simulink model "EPT"  (R2019b)
settings: Solver=FixedStepDiscrete  StartTime=0.0  StopTime=5  FixedStep=0.005  RelTol=1e-3  EnableMultiTasking=on
PreLoadFcn:
  | try, model_open; catch, disp('Error occurred while executing model pre-load callback: model_open.m'); disp('Please assure that the MATLAB working directory is set to the model directory before opening.'); end
InitFcn:
  | try, model_open; catch, end
undefined symbols (not defined in the file or in its folder): Bridge, GCM, H, ln, raptor_get_param_eval, raptor_get_safe_string, raptor_xcp_function
libraries: Raptor_lib x2810, simulink x374, hdlsllib x19
(part 39 of 45)

== system EPT/Foreground_TimeBase_5ms/CAN/CAN2_exec/ECHS/EPT2ECHS_TX/100ms_exec/0x1852FFF4_DBC ==
  note: Read_Actual_Torque
  Trigger : TriggerPort  VariantControl=Variant  PortDimensions=1
  Abs : Abs
  Constant : Constant  Value=8  OutDataTypeStr=uint8
  Constant1 : Constant  Value=0.01
  Constant2 : Constant  Value=0.02
  Convert_Data2Byte : Subsystem
  Convert_Data2Byte1 : Subsystem
  Data Type Conversion{,2..3,7..10} (7 alike) : DataTypeConversion
  Data Type Conversion{1,4..6} (4 alike) : DataTypeConversion  OutDataTypeStr=uint8
  Mux : Mux  Inputs=8
  raptor_adjustment7 : Raptor_lib/Data Storage/raptor_adjustment  paramName='EPT2ECHS_IV_TxID'  nameSource=Parameter  initValue=hex2dec('25')  dataType=uint32  storage=Calibration  calDispType=Number  calEnum={'False', 'True'}  calGain=1.0  calOffset=0.0  calMax=inf  calMin=-inf  calFormat='-1'  calUnit=''  calHelp=''  calAccess=1  calFunction=raptor_xcp_function(gcb)  calDispHeaders=off  calColHeaders={'Col1' 'Col2' 'Col3'}  calRowHeaders={'Row1' 'Row2' 'Row3'}
      settings: SourceProductName=Raptor
  raptor_can_txmsg : Raptor_lib/CAN/raptor_can_txmsg  canDefinition=struct('dbcFile', 'EPTvsECHS_V1.dbc','message', 'Display_Info_G3_Motor_MCU','comment', '','signals', {{'EPT_MOTOR_FAULT','EPT_MCU_OVERTEMP','EPT_MOTOR_OVERTEMP','EPT_MCU_TEMP','EPT_MOTOR_TEMP','EPT_MOTOR_TRQ','EPT_MOTOR_SPD'}},'enabled', [ 1 1 1 1 1 1 1;],'canBus', '''CAN2''','messageID', [ 408092660;],'idMask', [ 536870911;],'payloadMask', [],'payloadValue', [],'period', [ 0;],'mailbox', '','queueSize', [ 1;],'label', [ 1;],'ver', [ 2;],'showID', [ 0;],'showRaw', [ 0;],'fill', [ 0;],'editID', [ 0;],'signalOrder', [ 2;],'signalAscDes', [ 1;])  canBus='CAN2'  queueSize=1  payloadMask=[]  payloadValue=[]  period=0  showID=0  label=1  idMask=hex2dec('1FFFFFFF')  fill=0  id=408092660  showRaw=0  signalOrder=2  signalInfo={{struct('Name', 'EPT_MOTOR_OVERTEMP','Startbit', [ 0;],'SignalSize', [ 1;],'ByteOrder', 'LittleEndian','ValueType', 'UNSIGNED','Class', 'uint8','Signed', [ 0;],'Factor', [ 1;],'Offset', [ 0;],'Min', [ 0;],'Max', [ 0;],'Units', '','Comment', '','StartBit', [ 40;]),struct('Name', 'EPT_MOTOR_FAULT','Startbit', [ 0;],'SignalSize', [ 1;],'ByteOrder', 'LittleEndian','ValueType', 'UNSIGNED','Class', 'uint8','Signed', [ 0;],'Factor', [ 1;],'Offset', [ 0;],'Min', [ 0;],'Max', [ 0;],'Units', '','Comment', '','StartBit', [ 42;]),struct('Name', 'EPT_MCU_OVERTEMP','Startbit', [ 0;],'SignalSize', [ 1;],'ByteOrder', 'LittleEndian','ValueType', 'UNSIGNED','Class', 'uint8','Signed', [ 0;],'Factor', [ 1;],'Offset', [ 0;],'Min', [ 0;],'Max', [ 0;],'Units', '','Comment', '','StartBit', [ 41;]),struct('Name', 'EPT_MOTOR_TRQ','Startbit', [ 0;],'SignalSize', [ 8;],'ByteOrder', 'LittleEndian','ValueType', 'UNSIGNED','Class', 'uint8','Signed', [ 0;],'Factor', [ 0.4;],'Offset', [ 0;],'Min', [ 0;],'Max', [ 0;],'Units', '%','Comment', '','StartBit', [ 16;]),struct('Name', 'EPT_MOTOR_SPD','Startbit', [ 0;],'SignalSize', [ 16;],'ByteOrder', 'LittleEndian','ValueType', 'UNSIGNED','Class', 'uint16','Signed', [ 0;],'Factor', [ 1;],'Offset', [ 0;],'Min', [ 0;],'Max', [ 8000;],'Units', 'rpm','Comment', '','StartBit', [ 0;]),struct('Name', 'EPT_MCU_TEMP','Startbit', [ 0;],'SignalSize', [ 8;],'ByteOrder', 'LittleEndian','ValueType', 'UNSIGNED','Class', 'uint8','Signed', [ 0;],'Factor', [ 1;],'Offset', [ -40;],'Min', [ 0;],'Max', [ 100;],'Units', '℃','Comment', '','StartBit', [ 32;]),struct('Name', 'EPT_MOTOR_TEMP','Startbit', [ 0;],'SignalSize', [ 8;],'ByteOrder', 'LittleEndian','ValueType', 'UNSIGNED','Class', 'uint8','Signed', [ 0;],'Factor', [ 1;],'Offset', [ -40;],'Min', [ 0;],'Max', [ 100;],'Units', '℃','Comment', '','StartBit', [ 24;])}}
      settings: SourceProductName=Raptor
  raptor_can_txraw : Raptor_lib/CAN/raptor_can_txraw  canBus='CAN2'  queueSize=1  showIdTypePort=0  idTypeSelectValues=Standard|Extended  idTypeSelect=Standard
      settings: SourceProductName=Raptor
  raptor_data_def1 : Raptor_lib/Data Storage/raptor_data_def  dataName='EPT_MOTOR_TRQ'  initValue=0  dataType=double  storage=Volatile (RAM)  calVisible=on  calType=Measurement  calDispType=Number  calEnum={'False', 'True'}  calGain=1.0  calOffset=0  calMin=-inf  calMax=inf  calFormat='-1'  calUnit=''  calHelp=''  calAccess=1  calFunction=raptor_xcp_function(gcb)  calDispHeaders=off  calColHeaders={'Col1' 'Col2' 'Col3'}  calRowHeaders={'Row1' 'Row2' 'Row3'}
      settings: SourceProductName=Raptor
  raptor_data_def2 : Raptor_lib/Data Storage/raptor_data_def  dataName='EPT_MOTOR_FAULT'  initValue=0  dataType=boolean  storage=Volatile (RAM)  calVisible=on  calType=Measurement  calDispType=Number  calEnum={'False', 'True'}  calGain=1.0  calOffset=0  calMin=-inf  calMax=inf  calFormat='-1'  calUnit=''  calHelp=''  calAccess=1  calFunction=raptor_xcp_function(gcb)  calDispHeaders=off  calColHeaders={'Col1' 'Col2' 'Col3'}  calRowHeaders={'Row1' 'Row2' 'Row3'}
      settings: SourceProductName=Raptor
  raptor_data_def3 : Raptor_lib/Data Storage/raptor_data_def  dataName='EPT_MOTOR_SPD_DUP'  initValue=0  dataType=double  storage=Volatile (RAM)  calVisible=on  calType=Measurement  calDispType=Number  calEnum={'False', 'True'}  calGain=1.0  calOffset=0  calMin=-inf  calMax=inf  calFormat='-1'  calUnit=''  calHelp=''  calAccess=1  calFunction=raptor_xcp_function(gcb)  calDispHeaders=off  calColHeaders={'Col1' 'Col2' 'Col3'}  calRowHeaders={'Row1' 'Row2' 'Row3'}
      settings: SourceProductName=Raptor
  raptor_data_read1 : Raptor_lib/Data Storage/raptor_data_read  dataName='EPT_BPOBU_CURR'  dataShape=Scalar  idxSource=Input  idxRow=1  idxCol=1
      settings: SourceProductName=Raptor
  raptor_data_read11 : Raptor_lib/Data Storage/raptor_data_read  dataName='EPT_MOTOR_TRQ'  dataShape=Scalar  idxSource=Input  idxRow=1  idxCol=1
      settings: SourceProductName=Raptor
  raptor_data_read2 : Raptor_lib/Data Storage/raptor_data_read  dataName='EPT_MOTOR_SPD_DUP'  dataShape=Scalar  idxSource=Input  idxRow=1  idxCol=1
      settings: SourceProductName=Raptor
  raptor_data_read3 : Raptor_lib/Data Storage/raptor_data_read  dataName='Warning_Temperature_MCU_High'  dataShape=Scalar  idxSource=Input  idxRow=1  idxCol=1
      settings: SourceProductName=Raptor
  raptor_data_read4 : Raptor_lib/Data Storage/raptor_data_read  dataName='Fault_Temperature_Motor_High'  dataShape=Scalar  idxSource=Input  idxRow=1  idxCol=1
      settings: SourceProductName=Raptor
  raptor_data_read5 : Raptor_lib/Data Storage/raptor_data_read  dataName='EPT_BPOBU_VOLT'  dataShape=Scalar  idxSource=Input  idxRow=1  idxCol=1
      settings: SourceProductName=Raptor
  raptor_data_read6 : Raptor_lib/Data Storage/raptor_data_read  dataName='Read_Motor_Temp'  dataShape=Scalar  idxSource=Input  idxRow=1  idxCol=1
      settings: SourceProductName=Raptor
  raptor_data_read7 : Raptor_lib/Data Storage/raptor_data_read  dataName='Read_Motor_Speed'  dataShape=Scalar  idxSource=Input  idxRow=1  idxCol=1
      settings: SourceProductName=Raptor
  raptor_data_read8 : Raptor_lib/Data Storage/raptor_data_read  dataName='Read_Controller_Temp'  dataShape=Scalar  idxSource=Input  idxRow=1  idxCol=1
      settings: SourceProductName=Raptor
  raptor_data_read9 : Raptor_lib/Data Storage/raptor_data_read  dataName='EPT_MOTOR_FAULT'  dataShape=Scalar  idxSource=Input  idxRow=1  idxCol=1
      settings: SourceProductName=Raptor
  raptor_data_write17 : Raptor_lib/Data Storage/raptor_data_write  dataName='EPT_MOTOR_SPD_DUP'  dataShape=Scalar  idxSource=Input Port  idxRow=1  idxCol=1
      settings: SourceProductName=Raptor
  wires:
  raptor_data_read6/1 -> Data Type Conversion/1
  raptor_data_read8/1 -> Data Type Conversion3/1
  Mux/1 -> raptor_can_txraw/3
  Convert_Data2Byte/1(HighByte) -> Data Type Conversion1/1
  Convert_Data2Byte/2(LowByte) -> Data Type Conversion6/1
  Constant/1 -> raptor_can_txraw/2
  raptor_adjustment7/1 -> raptor_can_txraw/1
  Convert_Data2Byte1/1(HighByte) -> Data Type Conversion5/1
  Convert_Data2Byte1/2(LowByte) -> Data Type Conversion4/1
  raptor_data_read5/1 -> Convert_Data2Byte/1(Data)
  raptor_data_read1/1 -> Convert_Data2Byte1/1(Data)
  Constant1/1 -> Convert_Data2Byte/2(Factor)
  Constant2/1 -> Convert_Data2Byte1/2(Factor)
  Data Type Conversion1/1 -> Mux/3
  Data Type Conversion4/1 -> Mux/6
  Data Type Conversion5/1 -> Mux/5
  Data Type Conversion6/1 -> Mux/4
  raptor_data_read11/1 -> Data Type Conversion8/1
  Data Type Conversion8/1 -> raptor_can_txmsg/6  "EPT_MOTOR_TRQ"
  Data Type Conversion/1 -> raptor_can_txmsg/5  "EPT_MOTOR_TEMP"
  Abs/1 -> Data Type Conversion7/1
  Data Type Conversion7/1 -> raptor_data_write17/1
  raptor_data_read2/1 -> raptor_can_txmsg/7  "EPT_MOTOR_SPD"
  raptor_data_read7/1 -> Abs/1
  raptor_data_read4/1 -> Data Type Conversion9/1
  raptor_data_read3/1 -> Data Type Conversion2/1
  Data Type Conversion3/1 -> raptor_can_txmsg/4  "EPT_MCU_TEMP"
  Data Type Conversion2/1 -> raptor_can_txmsg/2  "EPT_MCU_OVERTEMP"
  Data Type Conversion9/1 -> raptor_can_txmsg/3  "EPT_MOTOR_OVERTEMP"
  Data Type Conversion10/1 -> raptor_can_txmsg/1  "EPT_MOTOR_FAULT"
  raptor_data_read9/1 -> Data Type Conversion10/1

== system EPT/Foreground_TimeBase_5ms/CAN/CAN2_exec/ECHS/EPT2ECHS_TX/100ms_exec/0x1853FFF4_DBC ==
  Trigger : TriggerPort  VariantControl=Variant  PortDimensions=1
  raptor_can_txmsg : Raptor_lib/CAN/raptor_can_txmsg  canDefinition=struct('dbcFile', 'EPTvsECHS_V1.dbc','message', 'Display_Info_G4_ESS_BPSWU','comment', '','signals', {{'EPT_PWCU_FAULT','EPT_BPSWU_SWAP_RMND','EPT_BPSWU_STA','EPT_PWCU_OUT_PWR','EPT_PWCU_TEMP','EPT_BPSWU_SOC','EPT_BPSWU_FCAP','EPT_BPSWU_NUM'}},'enabled', [ 1 1 1 1 1 1 1 1;],'canBus', '''CAN2''','messageID', [ 408158196;],'idMask', [ 536870911;],'payloadMask', [],'payloadValue', [],'period', [ 0;],'mailbox', '','queueSize', [ 1;],'label', [ 1;],'ver', [ 2;],'showID', [ 0;],'showRaw', [ 0;],'fill', [ 0;],'editID', [ 0;],'signalOrder', [ 2;],'signalAscDes', [ 1;])  canBus='CAN2'  queueSize=1  payloadMask=[]  payloadValue=[]  period=0  showID=0  label=1  idMask=hex2dec('1FFFFFFF')  fill=0  id=408158196  showRaw=0  signalOrder=2  signalInfo={{struct('Name', 'EPT_PWCU_TEMP','Startbit', [ 0;],'SignalSize', [ 8;],'ByteOrder', 'LittleEndian','ValueType', 'UNSIGNED','Class', 'uint8','Signed', [ 0;],'Factor', [ 1;],'Offset', [ -40;],'Min', [ 0;],'Max', [ 0;],'Units', '°C','Comment', '','StartBit', [ 24;]),struct('Name', 'EPT_PWCU_OUT_PWR','Startbit', [ 0;],'SignalSize', [ 8;],'ByteOrder', 'LittleEndian','ValueType', 'UNSIGNED','Class', 'uint8','Signed', [ 0;],'Factor', [ 0.1;],'Offset', [ 0;],'Min', [ 0;],'Max', [ 0;],'Units', 'Kw','Comment', '','StartBit', [ 32;]),struct('Name', 'EPT_PWCU_FAULT','Startbit', [ 0;],'SignalSize', [ 1;],'ByteOrder', 'LittleEndian','ValueType', 'UNSIGNED','Class', 'uint8','Signed', [ 0;],'Factor', [ 1;],'Offset', [ 0;],'Min', [ 0;],'Max', [ 0;],'Units', '','Comment', '','StartBit', [ 48;]),struct('Name', 'EPT_BPSWU_SWAP_RMND','Startbit', [ 0;],'SignalSize', [ 4;],'ByteOrder', 'LittleEndian','ValueType', 'UNSIGNED','Class', 'uint8','Signed', [ 0;],'Factor', [ 1;],'Offset', [ 0;],'Min', [ 0;],'Max', [ 0;],'Units', '','Comment', '','StartBit', [ 44;]),struct('Name', 'EPT_BPSWU_STA','Startbit', [ 0;],'SignalSize', [ 4;],'ByteOrder', 'LittleEndian','ValueType', 'UNSIGNED','Class', 'uint8','Signed', [ 0;],'Factor', [ 1;],'Offset', [ 0;],'Min', [ 0;],'Max', [ 0;],'Units', '','Comment', '','StartBit', [ 40;]),struct('Name', 'EPT_BPSWU_SOC','Startbit', [ 0;],'SignalSize', [ 8;],'ByteOrder', 'LittleEndian','ValueType', 'UNSIGNED','Class', 'uint8','Signed', [ 0;],'Factor', [ 0.5;],'Offset', [ 0;],'Min', [ 0;],'Max', [ 0;],'Units', '%','Comment', '','StartBit', [ 16;]),struct('Name', 'EPT_BPSWU_NUM','Startbit', [ 0;],'SignalSize', [ 4;],'ByteOrder', 'LittleEndian','ValueType', 'UNSIGNED','Class', 'uint8','Signed', [ 0;],'Factor', [ 1;],'Offset', [ 0;],'Min', [ 0;],'Max', [ 0;],'Units', '','Comment', '','StartBit', [ 0;]),struct('Name', 'EPT_BPSWU_FCAP','Startbit', [ 0;],'SignalSize', [ 8;],'ByteOrder', 'LittleEndian','ValueType', 'UNSIGNED','Class', 'uint8','Signed', [ 0;],'Factor', [ 0.4;],'Offset', [ 0;],'Min', [ 0;],'Max', [ 0;],'Units', '%','Comment', '','StartBit', [ 8;])}}
      settings: SourceProductName=Raptor

== system EPT/Foreground_TimeBase_5ms/CAN/CAN2_exec/ECHS/EPT2ECHS_TX/100ms_exec/CountTrigger ==
  Counter : Inport
  Constant1 : Constant  Value=0
  Constant3 : Constant
  CycleTrigger : Subsystem
  Switch : Switch  Threshold=1
  Unit Delay : UnitDelay  SampleTime=-1  HasFrameUpgradeWarning=on
  Tirgger : Outport  VectorParamsAs1DForOutWhenUnconnected=off
  wires:
  Unit Delay/1 -> Switch/2
  CycleTrigger/1(Trigger) -> Unit Delay/1, Tirgger/1
  Counter/1 -> CycleTrigger/2(In2)
  Constant1/1 -> Switch/1
  Constant3/1 -> Switch/3
  Switch/1 -> CycleTrigger/1(In1)

== system EPT/Foreground_TimeBase_5ms/CAN/CAN2_exec/ECHS/EPT2ECHS_TX/10ms_exec/0xC10D0F4_DBC ==
  note: Notes :
      | -EPT 2 ECHS Mode Enable
  Data Type Conversion1 : DataTypeConversion
  EPT_BPOBU_STA : Subsystem
  EPT_EW : Subsystem
  EPT_VEH_MODE_STA : Subsystem
  raptor_can_txmsg : Raptor_lib/CAN/raptor_can_txmsg  canDefinition=struct('dbcFile', 'EPTvsECHS_V1.dbc','message', 'EPT_Feedback_Status','comment', '','signals', {{'EPT_STATUS','EPT_VEH_MODE_STA','EPT_ERROR','EPT_BPOBU_STA','EPT_MAX_DRV_TRQ','EPT_MAX_REG_TRQ','EPT_CONSUMED_WH','EPT_MOTOR_SPD','EPT_GEAR_STA','EPT_CHG_REQ'}},'enabled', [ 1 1 1 1 1 1 1 1 1 1;],'canBus', '''CAN2''','messageID', [ 202428660;],'idMask', [ 536870911;],'payloadMask', [],'payloadValue', [],'period', [ 0;],'mailbox', '','queueSize', [ 1;],'label', [ 1;],'ver', [ 2;],'showID', [ 0;],'showRaw', [ 0;],'fill', [ 0;],'editID', [ 0;],'signalOrder', [ 2;])  canBus='CAN2'  queueSize=1  payloadMask=[]  payloadValue=[]  period=0  showID=0  label=1  idMask=hex2dec('1FFFFFFF')  fill=0  id=202428660  showRaw=0  signalOrder=2  signalInfo={{struct('Name', 'EPT_CHG_REQ','Startbit', [ 0;],'SignalSize', [ 1;],'ByteOrder', 'LittleEndian','ValueType', 'UNSIGNED','Class', 'uint8','Signed', [ 0;],'Factor', [ 1;],'Offset', [ 0;],'Min', [ 0;],'Max', [ 0;],'Units', '','Comment', '','StartBit', [ 63;]),struct('Name', 'EPT_BPOBU_STA','Startbit', [ 0;],'SignalSize', [ 3;],'ByteOrder', 'LittleEndian','ValueType', 'UNSIGNED','Class', 'uint8','Signed', [ 0;],'Factor', [ 1;],'Offset', [ 0;],'Min', [ 0;],'Max', [ 0;],'Units', '','Comment', '','StartBit', [ 5;]),struct('Name', 'EPT_GEAR_STA','Startbit', [ 0;],'SignalSize', [ 4;],'ByteOrder', 'LittleEndian','ValueType', 'UNSIGNED','Class', 'uint8','Signed', [ 0;],'Factor', [ 1;],'Offset', [ 0;],'Min', [ 0;],'Max', [ 0;],'Units', '','Comment', '','StartBit', [ 56;]),struct('Name', 'EPT_CONSUMED_WH','Startbit', [ 0;],'SignalSize', [ 16;],'ByteOrder', 'LittleEndian','ValueType', 'UNSIGNED','Class', 'uint16','Signed', [ 0;],'Factor', [ 1;],'Offset', [ 0;],'Min', [ 0;],'Max', [ 0;],'Units', 'WH','Comment', '','StartBit', [ 24;]),struct('Name', 'EPT_MAX_REG_TRQ','Startbit', [ 0;],'SignalSize', [ 8;],'ByteOrder', 'LittleEndian','ValueType', 'UNSIGNED','Class', 'uint8','Signed', [ 0;],'Factor', [ 1;],'Offset', [ 0;],'Min', [ 0;],'Max', [ 150;],'Units', 'Nm','Comment', '','StartBit', [ 16;]),struct('Name', 'EPT_MOTOR_SPD','Startbit', [ 0;],'SignalSize', [ 16;],'ByteOrder', 'LittleEndian','ValueType', 'UNSIGNED','Class', 'uint16','Signed', [ 0;],'Factor', [ 1;],'Offset', [ -12000;],'Min', [ -12000;],'Max', [ 12000;],'Units', 'rpm','Comment', '','StartBit', [ 40;]),struct('Name', 'EPT_STATUS','Startbit', [ 0;],'SignalSize', [ 1;],'ByteOrder', 'LittleEndian','ValueType', 'UNSIGNED','Class', 'uint8','Signed', [ 0;],'Factor', [ 1;],'Offset', [ 0;],'Min', [ 0;],'Max', [ 0;],'Units', '','Comment', '','StartBit', [ 0;]),struct('Name', 'EPT_VEH_MODE_STA','Startbit', [ 0;],'SignalSize', [ 2;],'ByteOrder', 'LittleEndian','ValueType', 'UNSIGNED','Class', 'uint8','Signed', [ 0;],'Factor', [ 1;],'Offset', [ 0;],'Min', [ 0;],'Max', [ 0;],'Units', '','Comment', '','StartBit', [ 1;]),struct('Name', 'EPT_ERROR','Startbit', [ 0;],'SignalSize', [ 2;],'ByteOrder', 'LittleEndian','ValueType', 'UNSIGNED','Class', 'uint8','Signed', [ 0;],'Factor', [ 1;],'Offset', [ 0;],'Min', [ 0;],'Max', [ 0;],'Units', '','Comment', '','StartBit', [ 3;]),struct('Name', 'EPT_MAX_DRV_TRQ','Startbit', [ 0;],'SignalSize', [ 8;],'ByteOrder', 'LittleEndian','ValueType', 'UNSIGNED','Class', 'uint8','Signed', [ 0;],'Factor', [ 1;],'Offset', [ 0;],'Min', [ 0;],'Max', [ 150;],'Units', 'Nm','Comment', '','StartBit', [ 8;])}}
      settings: SourceProductName=Raptor
  raptor_data_def1 : Raptor_lib/Data Storage/raptor_data_def  dataName='EPT_READY'  initValue=0  dataType=uint8  storage=Volatile (RAM)  calVisible=on  calType=Measurement  calDispType=Number  calEnum={'False', 'True'}  calGain=1.0  calOffset=0  calMin=-inf  calMax=inf  calFormat='-1'  calUnit=''  calHelp=''  calAccess=1  calFunction=raptor_xcp_function(gcb)  calDispHeaders=off  calColHeaders={'Col1' 'Col2' 'Col3'}  calRowHeaders={'Row1' 'Row2' 'Row3'}
      settings: SourceProductName=Raptor
  raptor_data_def2 : Raptor_lib/Data Storage/raptor_data_def  dataName='EPT_EW'  initValue=0  dataType=uint8  storage=Volatile (RAM)  calVisible=on  calType=Measurement  calDispType=Number  calEnum={'False', 'True'}  calGain=1.0  calOffset=0  calMin=-inf  calMax=inf  calFormat='-1'  calUnit=''  calHelp=''  calAccess=1  calFunction=raptor_xcp_function(gcb)  calDispHeaders=off  calColHeaders={'Col1' 'Col2' 'Col3'}  calRowHeaders={'Row1' 'Row2' 'Row3'}
      settings: SourceProductName=Raptor
  raptor_data_def3 : Raptor_lib/Data Storage/raptor_data_def  dataName='EPT_MAX_REG_TRQ'  initValue=0  dataType=double  storage=Volatile (RAM)  calVisible=on  calType=Measurement  calDispType=Number  calEnum={'False', 'True'}  calGain=1.0  calOffset=0  calMin=-inf  calMax=inf  calFormat='-1'  calUnit=''  calHelp=''  calAccess=1  calFunction=raptor_xcp_function(gcb)  calDispHeaders=off  calColHeaders={'Col1' 'Col2' 'Col3'}  calRowHeaders={'Row1' 'Row2' 'Row3'}
      settings: SourceProductName=Raptor
  raptor_data_def33 : Raptor_lib/Data Storage/raptor_data_def  dataName='EPT_VEH_MODE_STA'  initValue=0  dataType=uint8  storage=Volatile (RAM)  calVisible=on  calType=Measurement  calDispType=Number  calEnum={'False', 'True'}  calGain=1.0  calOffset=0  calMin=-inf  calMax=inf  calFormat='-1'  calUnit=''  calHelp=''  calAccess=1  calFunction=raptor_xcp_function(gcb)  calDispHeaders=off  calColHeaders={'Col1' 'Col2' 'Col3'}  calRowHeaders={'Row1' 'Row2' 'Row3'}
      settings: SourceProductName=Raptor
  raptor_data_def34 : Raptor_lib/Data Storage/raptor_data_def  dataName='EPT_MAX_DRV_TRQ'  initValue=0  dataType=double  storage=Volatile (RAM)  calVisible=on  calType=Measurement  calDispType=Number  calEnum={'False', 'True'}  calGain=1.0  calOffset=0  calMin=-inf  calMax=inf  calFormat='-1'  calUnit=''  calHelp=''  calAccess=1  calFunction=raptor_xcp_function(gcb)  calDispHeaders=off  calColHeaders={'Col1' 'Col2' 'Col3'}  calRowHeaders={'Row1' 'Row2' 'Row3'}
      settings: SourceProductName=Raptor
  raptor_data_def4 : Raptor_lib/Data Storage/raptor_data_def  dataName='EPT_MOTOR_SPD'  initValue=0  dataType=int16  storage=Volatile (RAM)  calVisible=on  calType=Measurement  calDispType=Number  calEnum={'False', 'True'}  calGain=1.0  calOffset=0  calMin=-inf  calMax=inf  calFormat='-1'  calUnit=''  calHelp=''  calAccess=1  calFunction=raptor_xcp_function(gcb)  calDispHeaders=off  calColHeaders={'Col1' 'Col2' 'Col3'}  calRowHeaders={'Row1' 'Row2' 'Row3'}
      settings: SourceProductName=Raptor
  raptor_data_def5 : Raptor_lib/Data Storage/raptor_data_def  dataName='EPT_CONSUMED_WH'  initValue=0  dataType=double  storage=Volatile (RAM)  calVisible=on  calType=Measurement  calDispType=Number  calEnum={'False', 'True'}  calGain=1.0  calOffset=0  calMin=-inf  calMax=inf  calFormat='-1'  calUnit=''  calHelp=''  calAccess=1  calFunction=raptor_xcp_function(gcb)  calDispHeaders=off  calColHeaders={'Col1' 'Col2' 'Col3'}  calRowHeaders={'Row1' 'Row2' 'Row3'}
      settings: SourceProductName=Raptor
  raptor_data_def6 : Raptor_lib/Data Storage/raptor_data_def  dataName='EPT_BPOBU_STA'  initValue=0  dataType=double  storage=Volatile (RAM)  calVisible=on  calType=Measurement  calDispType=Number  calEnum={'False', 'True'}  calGain=1.0  calOffset=0  calMin=-inf  calMax=inf  calFormat='-1'  calUnit=''  calHelp=''  calAccess=1  calFunction=raptor_xcp_function(gcb)  calDispHeaders=off  calColHeaders={'Col1' 'Col2' 'Col3'}  calRowHeaders={'Row1' 'Row2' 'Row3'}
      settings: SourceProductName=Raptor
  raptor_data_def7 : Raptor_lib/Data Storage/raptor_data_def  dataName='EPT_GEAR_STA'  initValue=0  dataType=int16  storage=Volatile (RAM)  calVisible=on  calType=Measurement  calDispType=Number  calEnum={'False', 'True'}  calGain=1.0  calOffset=0  calMin=-inf  calMax=inf  calFormat='-1'  calUnit=''  calHelp=''  calAccess=1  calFunction=raptor_xcp_function(gcb)  calDispHeaders=off  calColHeaders={'Col1' 'Col2' 'Col3'}  calRowHeaders={'Row1' 'Row2' 'Row3'}
      settings: SourceProductName=Raptor
  raptor_data_def8 : Raptor_lib/Data Storage/raptor_data_def  dataName='EPT_CHG_REQ'  initValue=0  dataType=boolean  storage=Volatile (RAM)  calVisible=on  calType=Measurement  calDispType=Number  calEnum={'False', 'True'}  calGain=1.0  calOffset=0  calMin=-inf  calMax=inf  calFormat='-1'  calUnit=''  calHelp=''  calAccess=1  calFunction=raptor_xcp_function(gcb)  calDispHeaders=off  calColHeaders={'Col1' 'Col2' 'Col3'}  calRowHeaders={'Row1' 'Row2' 'Row3'}
      settings: SourceProductName=Raptor
  raptor_data_read1 : Raptor_lib/Data Storage/raptor_data_read  dataName='EPT_READY'  dataShape=Scalar  idxSource=Input  idxRow=1  idxCol=1
      settings: SourceProductName=Raptor
  raptor_data_read10 : Raptor_lib/Data Storage/raptor_data_read  dataName='EPT_GEAR_STA'  dataShape=Scalar  idxSource=Input  idxRow=1  idxCol=1
      settings: SourceProductName=Raptor
  raptor_data_read11 : Raptor_lib/Data Storage/raptor_data_read  dataName='EPT_CHG_REQ'  dataShape=Scalar  idxSource=Input  idxRow=1  idxCol=1
      settings: SourceProductName=Raptor
  raptor_data_read2 : Raptor_lib/Data Storage/raptor_data_read  dataName='EPT_EW'  dataShape=Scalar  idxSource=Input  idxRow=1  idxCol=1
      settings: SourceProductName=Raptor
  raptor_data_read3 : Raptor_lib/Data Storage/raptor_data_read  dataName='EPT_MAX_DRV_TRQ'  dataShape=Scalar  idxSource=Input  idxRow=1  idxCol=1
      settings: SourceProductName=Raptor
  raptor_data_read4 : Raptor_lib/Data Storage/raptor_data_read  dataName='EPT_VEH_MODE_STA'  dataShape=Scalar  idxSource=Input  idxRow=1  idxCol=1
      settings: SourceProductName=Raptor
  raptor_data_read5 : Raptor_lib/Data Storage/raptor_data_read  dataName='EPT_MAX_REG_TRQ'  dataShape=Scalar  idxSource=Input  idxRow=1  idxCol=1
      settings: SourceProductName=Raptor
  raptor_data_read6 : Raptor_lib/Data Storage/raptor_data_read  dataName='EPT_MOTOR_SPD'  dataShape=Scalar  idxSource=Input  idxRow=1  idxCol=1
      settings: SourceProductName=Raptor
  raptor_data_read7 : Raptor_lib/Data Storage/raptor_data_read  dataName='Read_Motor_Speed'  dataShape=Scalar  idxSource=Input  idxRow=1  idxCol=1
      settings: SourceProductName=Raptor
  raptor_data_read8 : Raptor_lib/Data Storage/raptor_data_read  dataName='EPT_CONSUMED_WH'  dataShape=Scalar  idxSource=Input  idxRow=1  idxCol=1
      settings: SourceProductName=Raptor
  raptor_data_read9 : Raptor_lib/Data Storage/raptor_data_read  dataName='EPT_BPOBU_STA'  dataShape=Scalar  idxSource=Input  idxRow=1  idxCol=1
      settings: SourceProductName=Raptor
  raptor_data_write17 : Raptor_lib/Data Storage/raptor_data_write  dataName='EPT_MOTOR_SPD'  dataShape=Scalar  idxSource=Input Port  idxRow=1  idxCol=1
      settings: SourceProductName=Raptor
  wires:
  raptor_data_read10/1 -> raptor_can_txmsg/9  "EPT_GEAR_STA"
  raptor_data_read6/1 -> raptor_can_txmsg/8  "EPT_MOTOR_SPD"
  raptor_data_read8/1 -> raptor_can_txmsg/7  "EPT_CONSUMED_WH"
  raptor_data_read3/1 -> raptor_can_txmsg/5  "EPT_MAX_DRV_TRQ"
  raptor_data_read9/1 -> raptor_can_txmsg/4  "EPT_BPOBU_STA"
  raptor_data_read4/1 -> raptor_can_txmsg/2  "EPT_VEH_MODE_STA"
  raptor_data_read2/1 -> raptor_can_txmsg/3  "EPT_ERROR"
  raptor_data_read5/1 -> raptor_can_txmsg/6  "EPT_MAX_REG_TRQ"
  raptor_data_read1/1 -> raptor_can_txmsg/1  "EPT_STATUS"
  raptor_data_read11/1 -> raptor_can_txmsg/10  "EPT_CHG_REQ"
  raptor_data_read7/1 -> Data Type Conversion1/1
  Data Type Conversion1/1 -> raptor_data_write17/1

== system EPT/Foreground_TimeBase_5ms/CAN/CAN2_exec/ECHS/EPT2ECHS_TX/500ms_exec/0x1820FFF4_DBC ==
  Trigger : TriggerPort  VariantControl=Variant  PortDimensions=1
  raptor_can_txmsg : Raptor_lib/CAN/raptor_can_txmsg  canDefinition=struct('dbcFile', 'EPTvsECHS_V1.dbc','message', 'Remote_DA_Status_G20_ESS_OBU_1','comment', '','signals', {{'BP_OBU_Fault_G5','BP_OBU_Fault_G4','BP_OBU_Fault_G3','BP_OBU_Fault_G2','BP_OBU_Fault_G1','BP_OBU_Warning_G3','BP_OBU_Warning_G2','BP_OBU_Warning_G1'}},'enabled', [ 1 1 1 1 1 1 1 1;],'canBus', '''CAN2''','messageID', [ 404815860;],'idMask', [ 536870911;],'payloadMask', [],'payloadValue', [],'period', [ 0;],'mailbox', '','queueSize', [ 1;],'label', [ 0;],'ver', [ 2;],'showID', [ 0;],'showRaw', [ 0;],'fill', [ 0;],'editID', [ 0;],'signalOrder', [ 2;],'signalAscDes', [ 1;])  canBus='CAN2'  queueSize=1  payloadMask=[]  payloadValue=[]  period=0  showID=0  label=0  idMask=hex2dec('1FFFFFFF')  fill=0  id=404815860  showRaw=0  signalOrder=2  signalInfo={{struct('Name', 'BP_OBU_Warning_G3','Startbit', [ 0;],'SignalSize', [ 8;],'ByteOrder', 'LittleEndian','ValueType', 'UNSIGNED','Class', 'uint8','Signed', [ 0;],'Factor', [ 1;],'Offset', [ 0;],'Min', [ 0;],'Max', [ 0;],'Units', '','Comment', '','StartBit', [ 16;]),struct('Name', 'BP_OBU_Warning_G2','Startbit', [ 0;],'SignalSize', [ 8;],'ByteOrder', 'LittleEndian','ValueType', 'UNSIGNED','Class', 'uint8','Signed', [ 0;],'Factor', [ 1;],'Offset', [ 0;],'Min', [ 0;],'Max', [ 0;],'Units', '','Comment', '','StartBit', [ 8;]),struct('Name', 'BP_OBU_Warning_G1','Startbit', [ 0;],'SignalSize', [ 8;],'ByteOrder', 'LittleEndian','ValueType', 'UNSIGNED','Class', 'uint8','Signed', [ 0;],'Factor', [ 1;],'Offset', [ 0;],'Min', [ 0;],'Max', [ 0;],'Units', '','Comment', '','StartBit', [ 0;]),struct('Name', 'BP_OBU_Fault_G5','Startbit', [ 0;],'SignalSize', [ 8;],'ByteOrder', 'LittleEndian','ValueType', 'UNSIGNED','Class', 'uint8','Signed', [ 0;],'Factor', [ 1;],'Offset', [ 0;],'Min', [ 0;],'Max', [ 0;],'Units', '','Comment', '','StartBit', [ 56;]),struct('Name', 'BP_OBU_Fault_G4','Startbit', [ 0;],'SignalSize', [ 8;],'ByteOrder', 'LittleEndian','ValueType', 'UNSIGNED','Class', 'uint8','Signed', [ 0;],'Factor', [ 1;],'Offset', [ 0;],'Min', [ 0;],'Max', [ 0;],'Units', '','Comment', '','StartBit', [ 48;]),struct('Name', 'BP_OBU_Fault_G3','Startbit', [ 0;],'SignalSize', [ 8;],'ByteOrder', 'LittleEndian','ValueType', 'UNSIGNED','Class', 'uint8','Signed', [ 0;],'Factor', [ 1;],'Offset', [ 0;],'Min', [ 0;],'Max', [ 0;],'Units', '','Comment', '','StartBit', [ 40;]),struct('Name', 'BP_OBU_Fault_G2','Startbit', [ 0;],'SignalSize', [ 8;],'ByteOrder', 'LittleEndian','ValueType', 'UNSIGNED','Class', 'uint8','Signed', [ 0;],'Factor', [ 1;],'Offset', [ 0;],'Min', [ 0;],'Max', [ 0;],'Units', '','Comment', '','StartBit', [ 32;]),struct('Name', 'BP_OBU_Fault_G1','Startbit', [ 0;],'SignalSize', [ 8;],'ByteOrder', 'LittleEndian','ValueType', 'UNSIGNED','Class', 'uint8','Signed', [ 0;],'Factor', [ 1;],'Offset', [ 0;],'Min', [ 0;],'Max', [ 0;],'Units', '','Comment', '','StartBit', [ 24;])}}
      settings: SourceProductName=Raptor
  raptor_data_read1 : Raptor_lib/Data Storage/raptor_data_read  dataName='BP_OBU_Fault_G4'  dataShape=Scalar  idxSource=Input  idxRow=1  idxCol=1
      settings: SourceProductName=Raptor
  raptor_data_read2 : Raptor_lib/Data Storage/raptor_data_read  dataName='BP_OBU_Fault_G3'  dataShape=Scalar  idxSource=Input  idxRow=1  idxCol=1
      settings: SourceProductName=Raptor
  raptor_data_read3 : Raptor_lib/Data Storage/raptor_data_read  dataName='BP_OBU_Fault_G2'  dataShape=Scalar  idxSource=Input  idxRow=1  idxCol=1
      settings: SourceProductName=Raptor
  raptor_data_read4 : Raptor_lib/Data Storage/raptor_data_read  dataName='BP_OBU_Fault_G5'  dataShape=Scalar  idxSource=Input  idxRow=1  idxCol=1
      settings: SourceProductName=Raptor
  raptor_data_read5 : Raptor_lib/Data Storage/raptor_data_read  dataName='BP_OBU_Fault_G1'  dataShape=Scalar  idxSource=Input  idxRow=1  idxCol=1
      settings: SourceProductName=Raptor
  raptor_data_read6 : Raptor_lib/Data Storage/raptor_data_read  dataName='BP_OBU_Warning_G3'  dataShape=Scalar  idxSource=Input  idxRow=1  idxCol=1
      settings: SourceProductName=Raptor
  raptor_data_read7 : Raptor_lib/Data Storage/raptor_data_read  dataName='BP_OBU_Warning_G2'  dataShape=Scalar  idxSource=Input  idxRow=1  idxCol=1
      settings: SourceProductName=Raptor
  raptor_data_read8 : Raptor_lib/Data Storage/raptor_data_read  dataName='BP_OBU_Warning_G1'  dataShape=Scalar  idxSource=Input  idxRow=1  idxCol=1
      settings: SourceProductName=Raptor
  wires:
  raptor_data_read4/1 -> raptor_can_txmsg/1
  raptor_data_read1/1 -> raptor_can_txmsg/2
  raptor_data_read8/1 -> raptor_can_txmsg/8
  raptor_data_read7/1 -> raptor_can_txmsg/7
  raptor_data_read6/1 -> raptor_can_txmsg/6
  raptor_data_read5/1 -> raptor_can_txmsg/5
  raptor_data_read3/1 -> raptor_can_txmsg/4
  raptor_data_read2/1 -> raptor_can_txmsg/3

== system EPT/Foreground_TimeBase_5ms/CAN/CAN2_exec/ECHS/EPT2ECHS_TX/500ms_exec/CountTrigger ==
  Counter : Inport
  Constant1 : Constant  Value=0
  Constant3 : Constant
  CycleTrigger : Subsystem
  Switch : Switch  Threshold=1
  Unit Delay : UnitDelay  SampleTime=-1  HasFrameUpgradeWarning=on
  Tirgger : Outport  VectorParamsAs1DForOutWhenUnconnected=off
  wires:
  Switch/1 -> CycleTrigger/1(In1)
  Constant3/1 -> Switch/3
  Constant1/1 -> Switch/1
  Counter/1 -> CycleTrigger/2(In2)
  CycleTrigger/1(Trigger) -> Tirgger/1, Unit Delay/1
  Unit Delay/1 -> Switch/2

== system EPT/Foreground_TimeBase_5ms/CAN/CAN2_exec/IVT2/Coulomb Counting Method1/20ms/CountTrigger3 ==
  Counter : Inport
  Constant1 : Constant  Value=0
  Constant3 : Constant
  CycleTrigger : Subsystem
  Switch : Switch  Threshold=1
  Unit Delay1 : UnitDelay  SampleTime=-1  HasFrameUpgradeWarning=on
  Unit Delay2 : UnitDelay  SampleTime=-1  HasFrameUpgradeWarning=on
  Tirgger : Outport  VectorParamsAs1DForOutWhenUnconnected=off
  wires:
  Unit Delay2/1 -> Tirgger/1
  Unit Delay1/1 -> CycleTrigger/1(In1)
  CycleTrigger/1(Trigger) -> Unit Delay2/1, Switch/2
  Counter/1 -> CycleTrigger/2(In2)
  Constant1/1 -> Switch/1
  Constant3/1 -> Switch/3
  Switch/1 -> Unit Delay1/1

== system EPT/Foreground_TimeBase_5ms/CAN/CAN2_exec/IVT2/Coulomb Counting Method1/CountTrigger/CycleTrigger ==
  In1 : Inport
  In2 : Inport  Port=2
  Add : Sum
  Add2 : Sum  Inputs=+-
  Constant2 : Constant  Value=0
  Constant3 : Constant
  Data Type Conversion1 : DataTypeConversion
  Data Type Conversion2 : DataTypeConversion
  Relational Operator1 : RelationalOperator  OutDataTypeStr=boolean  RndMeth=Simplest
  Scope1 : Scope
  Scope2 : Scope
  Switch : Switch  Threshold=1
  Unit Delay : UnitDelay  SampleTime=-1  HasFrameUpgradeWarning=on
  Trigger : Outport  VectorParamsAs1DForOutWhenUnconnected=off
  wires:
  Constant3/1 -> Add2/2
  In2/1 -> Add2/1
  Add2/1 -> Data Type Conversion1/1
  Data Type Conversion2/1 -> Switch/2, Add/2
  Constant2/1 -> Switch/3
  Data Type Conversion1/1 -> Relational Operator1/2
  Relational Operator1/1 -> Trigger/1, Scope2/1
  Switch/1 -> Unit Delay/1, Scope1/1, Relational Operator1/1
  Unit Delay/1 -> Add/1
  In1/1 -> Data Type Conversion2/1
  Add/1 -> Switch/1

== system EPT/Foreground_TimeBase_5ms/CAN/CAN3_exec/OBC/OBC/OBC_Rx/Convert_Byte2Data1 ==
  HighByte : Inport
  LowByte : Inport  Port=2
  Offset : Inport  Port=3
  Factor : Inport  Port=4
  Add2 : Sum
  Add5 : Sum
  Constant10 : Constant  Value=256
  Data Type Conversion10 : DataTypeConversion  OutDataTypeStr=double
  Divide6 : Product  Inputs=**
  Divide9 : Product  Inputs=**
  Data : Outport  VectorParamsAs1DForOutWhenUnconnected=off
  wires:
  Divide6/1 -> Add2/2
  LowByte/1 -> Add2/1
  Add5/1 -> Data Type Conversion10/1
  HighByte/1 -> Divide6/1
  Constant10/1 -> Divide6/2
  Divide9/1 -> Add5/1
  Add2/1 -> Divide9/1
  Data Type Conversion10/1 -> Data/1
  Factor/1 -> Divide9/2
  Offset/1 -> Add5/2

== system EPT/Foreground_TimeBase_5ms/CAN/CAN3_exec/OBC/OBC/OBC_Rx/Convert_Byte2Data2 ==
  HighByte : Inport
  LowByte : Inport  Port=2
  Offset : Inport  Port=3
  Factor : Inport  Port=4
  Add2 : Sum
  Add5 : Sum
  Constant10 : Constant  Value=256
  Data Type Conversion10 : DataTypeConversion  OutDataTypeStr=double
  Divide6 : Product  Inputs=**
  Divide9 : Product  Inputs=**
  Data : Outport  VectorParamsAs1DForOutWhenUnconnected=off
  wires:
  Divide6/1 -> Add2/2
  LowByte/1 -> Add2/1
  Add5/1 -> Data Type Conversion10/1
  HighByte/1 -> Divide6/1
  Constant10/1 -> Divide6/2
  Divide9/1 -> Add5/1
  Add2/1 -> Divide9/1
  Data Type Conversion10/1 -> Data/1
  Factor/1 -> Divide9/2
  Offset/1 -> Add5/2

== system EPT/Foreground_TimeBase_5ms/CAN/CAN3_exec/OBC/OBC/OBC_Rx/Convert_Byte2Data3 ==
  HighByte : Inport
  LowByte : Inport  Port=2
  Offset : Inport  Port=3
  Factor : Inport  Port=4
  Add2 : Sum
  Add5 : Sum
  Constant10 : Constant  Value=256
  Data Type Conversion10 : DataTypeConversion  OutDataTypeStr=double
  Divide6 : Product  Inputs=**
  Divide9 : Product  Inputs=**
  Data : Outport  VectorParamsAs1DForOutWhenUnconnected=off
  wires:
  Divide6/1 -> Add2/2
  LowByte/1 -> Add2/1
  Add5/1 -> Data Type Conversion10/1
  HighByte/1 -> Divide6/1
  Constant10/1 -> Divide6/2
  Divide9/1 -> Add5/1
  Add2/1 -> Divide9/1
  Data Type Conversion10/1 -> Data/1
  Factor/1 -> Divide9/2
  Offset/1 -> Add5/2

== system EPT/Foreground_TimeBase_5ms/CAN/CAN3_exec/OBC/OBC/OBC_Tx/Convert_Data2Byte ==
  Data : Inport
  Factor : Inport  Port=2
  Offset : Inport  Port=3
  Add1 : Sum
  Bitwise Operator : simulink/Logic and Bit Operations/Bitwise Operator  logicop=AND  UseBitMask=on  BitMask=bin2dec('1111111100000000')  BitMaskRealWorld=Stored Integer
  Bitwise Operator1 : simulink/Logic and Bit Operations/Bitwise Operator  logicop=AND  UseBitMask=on  BitMask=bin2dec('0000000011111111')  BitMaskRealWorld=Stored Integer
  Constant : Constant
  Data Type Conversion1 : DataTypeConversion  OutDataTypeStr=uint16
  Divide1 : Product  Inputs=*/
  Divide2 : Product  Inputs=**
  Shift Arithmetic : ArithShift  BitShiftNumber=8  BitShiftDirection=Right
  HighByte : Outport  VectorParamsAs1DForOutWhenUnconnected=off
  LowByte : Outport  Port=2  VectorParamsAs1DForOutWhenUnconnected=off
  wires:
  Divide2/1 -> Data Type Conversion1/1
  Data/1 -> Add1/1
  Add1/1 -> Divide2/1
  Data Type Conversion1/1 -> Bitwise Operator1/1, Bitwise Operator/1
  Bitwise Operator1/1 -> LowByte/1
  Shift Arithmetic/1 -> HighByte/1
  Offset/1 -> Add1/2
  Bitwise Operator/1 -> Shift Arithmetic/1
  Factor/1 -> Divide1/2
  Divide1/1 -> Divide2/2
  Constant/1 -> Divide1/1

== system EPT/Foreground_TimeBase_5ms/CAN/CAN3_exec/OBC/OBC/OBC_Tx/Convert_Data2Byte1 ==
  Data : Inport
  Factor : Inport  Port=2
  Offset : Inport  Port=3
  Add1 : Sum
  Bitwise Operator : simulink/Logic and Bit Operations/Bitwise Operator  logicop=AND  UseBitMask=on  BitMask=bin2dec('1111111100000000')  BitMaskRealWorld=Stored Integer
  Bitwise Operator1 : simulink/Logic and Bit Operations/Bitwise Operator  logicop=AND  UseBitMask=on  BitMask=bin2dec('0000000011111111')  BitMaskRealWorld=Stored Integer
  Constant : Constant
  Data Type Conversion1 : DataTypeConversion  OutDataTypeStr=uint16
  Divide1 : Product  Inputs=*/
  Divide2 : Product  Inputs=**
  Shift Arithmetic : ArithShift  BitShiftNumber=8  BitShiftDirection=Right
  HighByte : Outport  VectorParamsAs1DForOutWhenUnconnected=off
  LowByte : Outport  Port=2  VectorParamsAs1DForOutWhenUnconnected=off
  wires:
  Constant/1 -> Divide1/1
  Divide1/1 -> Divide2/2
  Factor/1 -> Divide1/2
  Bitwise Operator/1 -> Shift Arithmetic/1
  Offset/1 -> Add1/2
  Shift Arithmetic/1 -> HighByte/1
  Bitwise Operator1/1 -> LowByte/1
  Data Type Conversion1/1 -> Bitwise Operator/1, Bitwise Operator1/1
  Add1/1 -> Divide2/1
  Data/1 -> Add1/1
  Divide2/1 -> Data Type Conversion1/1

== system EPT/Foreground_TimeBase_5ms/CAN/CAN3_exec/PWCU_GENERATOR/PWCU/CountTrigger1/CycleTrigger ==
  In1 : Inport
  In2 : Inport  Port=2
  Add : Sum
  Add1 : Sum
  Add2 : Sum  Inputs=+-
  Constant1 : Constant
  Constant2 : Constant  Value=0
  Constant3 : Constant
  Data Type Conversion1 : DataTypeConversion
  Data Type Conversion2 : DataTypeConversion
  Display : Display
  Relational Operator1 : RelationalOperator  OutDataTypeStr=boolean  RndMeth=Simplest
  Scope : Scope
  Scope1 : Scope
  Scope2 : Scope
  Switch : Switch  Threshold=1
  Unit Delay : UnitDelay  SampleTime=-1  HasFrameUpgradeWarning=on
  Unit Delay1 : UnitDelay  SampleTime=-1  HasFrameUpgradeWarning=on
  Trigger : Outport  VectorParamsAs1DForOutWhenUnconnected=off
  wires:
  Constant3/1 -> Add2/2
  In2/1 -> Add2/1
  Add2/1 -> Data Type Conversion1/1
  Data Type Conversion2/1 -> Switch/2, Add/2
  Constant2/1 -> Switch/3
  Data Type Conversion1/1 -> Relational Operator1/2
  Relational Operator1/1 -> Trigger/1, Scope2/1
  Constant1/1 -> Add1/2
  Unit Delay1/1 -> Add1/1
  Add1/1 -> Display/1, Unit Delay1/1, Scope/1
  Switch/1 -> Unit Delay/1, Scope1/1, Relational Operator1/1
  Unit Delay/1 -> Add/1
  In1/1 -> Data Type Conversion2/1
  Add/1 -> Switch/1

== system EPT/Foreground_TimeBase_5ms/CAN/CAN3_exec/PWCU_GENERATOR/PWCU/PWCU 2_Rx/Convert_Byte2Data ==
  HighByte : Inport
  LowByte : Inport  Port=2
  Offset : Inport  Port=3
  Factor : Inport  Port=4
  Add2 : Sum
  Add5 : Sum
  Constant10 : Constant  Value=256
  Data Type Conversion10 : DataTypeConversion  OutDataTypeStr=double
  Divide6 : Product  Inputs=**
  Divide9 : Product  Inputs=**
  Data : Outport  VectorParamsAs1DForOutWhenUnconnected=off
  wires:
  Divide6/1 -> Add2/2
  LowByte/1 -> Add2/1
  Add5/1 -> Data Type Conversion10/1
  HighByte/1 -> Divide6/1
  Constant10/1 -> Divide6/2
  Divide9/1 -> Add5/1
  Add2/1 -> Divide9/1
  Data Type Conversion10/1 -> Data/1
  Factor/1 -> Divide9/2
  Offset/1 -> Add5/2

== system EPT/Foreground_TimeBase_5ms/CAN/CAN3_exec/PWCU_GENERATOR/PWCU/PWCU 2_Rx/Convert_Byte2Data1 ==
  HighByte : Inport
  LowByte : Inport  Port=2
  Offset : Inport  Port=3
  Factor : Inport  Port=4
  Add2 : Sum
  Add5 : Sum
  Constant10 : Constant  Value=256
  Data Type Conversion10 : DataTypeConversion  OutDataTypeStr=double
  Divide6 : Product  Inputs=**
  Divide9 : Product  Inputs=**
  Data : Outport  VectorParamsAs1DForOutWhenUnconnected=off
  wires:
  Divide6/1 -> Add2/2
  LowByte/1 -> Add2/1
  Add5/1 -> Data Type Conversion10/1
  HighByte/1 -> Divide6/1
  Constant10/1 -> Divide6/2
  Divide9/1 -> Add5/1
  Add2/1 -> Divide9/1
  Data Type Conversion10/1 -> Data/1
  Factor/1 -> Divide9/2
  Offset/1 -> Add5/2

== system EPT/Foreground_TimeBase_5ms/CAN/CAN3_exec/PWCU_GENERATOR/PWCU/PWCU 2_Rx/Convert_Byte2Data2 ==
  HighByte : Inport
  LowByte : Inport  Port=2
  Offset : Inport  Port=3
  Factor : Inport  Port=4
  Add2 : Sum
  Add5 : Sum
  Constant10 : Constant  Value=256
  Data Type Conversion10 : DataTypeConversion  OutDataTypeStr=double
  Divide6 : Product  Inputs=**
  Divide9 : Product  Inputs=**
  Data : Outport  VectorParamsAs1DForOutWhenUnconnected=off
  wires:
  Divide6/1 -> Add2/2
  LowByte/1 -> Add2/1
  Add5/1 -> Data Type Conversion10/1
  HighByte/1 -> Divide6/1
  Constant10/1 -> Divide6/2
  Divide9/1 -> Add5/1
  Add2/1 -> Divide9/1
  Data Type Conversion10/1 -> Data/1
  Factor/1 -> Divide9/2
  Offset/1 -> Add5/2

== system EPT/Foreground_TimeBase_5ms/CAN/CAN3_exec/PWCU_GENERATOR/PWCU/PWCU 3_Rx/Convert_Byte2Data ==
  HighByte : Inport
  LowByte : Inport  Port=2
  Offset : Inport  Port=3
  Factor : Inport  Port=4
  Add2 : Sum
  Add5 : Sum
  Constant10 : Constant  Value=256
  Data Type Conversion10 : DataTypeConversion  OutDataTypeStr=double
  Divide6 : Product  Inputs=**
  Divide9 : Product  Inputs=**
  Data : Outport  VectorParamsAs1DForOutWhenUnconnected=off
  wires:
  Offset/1 -> Add5/2
  Factor/1 -> Divide9/2
  Data Type Conversion10/1 -> Data/1
  Add2/1 -> Divide9/1
  Divide9/1 -> Add5/1
  Constant10/1 -> Divide6/2
  HighByte/1 -> Divide6/1
  Add5/1 -> Data Type Conversion10/1
  LowByte/1 -> Add2/1
  Divide6/1 -> Add2/2

== system EPT/Foreground_TimeBase_5ms/CAN/CAN3_exec/PWCU_GENERATOR/PWCU/PWCU 3_Rx/Convert_Byte2Data1 ==
  HighByte : Inport
  LowByte : Inport  Port=2
  Offset : Inport  Port=3
  Factor : Inport  Port=4
  Add2 : Sum
  Add5 : Sum
  Constant10 : Constant  Value=256
  Data Type Conversion10 : DataTypeConversion  OutDataTypeStr=double
  Divide6 : Product  Inputs=**
  Divide9 : Product  Inputs=**
  Data : Outport  VectorParamsAs1DForOutWhenUnconnected=off
  wires:
  Offset/1 -> Add5/2
  Factor/1 -> Divide9/2
  Data Type Conversion10/1 -> Data/1
  Add2/1 -> Divide9/1
  Divide9/1 -> Add5/1
  Constant10/1 -> Divide6/2
  HighByte/1 -> Divide6/1
  Add5/1 -> Data Type Conversion10/1
  LowByte/1 -> Add2/1
  Divide6/1 -> Add2/2

== system EPT/Foreground_TimeBase_5ms/CAN/CAN3_exec/PWCU_GENERATOR/PWCU/PWCU 3_Rx/Convert_Byte2Data2 ==
  HighByte : Inport
  LowByte : Inport  Port=2
  Offset : Inport  Port=3
  Factor : Inport  Port=4
  Add2 : Sum
  Add5 : Sum
  Constant10 : Constant  Value=256
  Data Type Conversion10 : DataTypeConversion  OutDataTypeStr=double
  Divide6 : Product  Inputs=**
  Divide9 : Product  Inputs=**
  Data : Outport  VectorParamsAs1DForOutWhenUnconnected=off
  wires:
  Offset/1 -> Add5/2
  Factor/1 -> Divide9/2
  Data Type Conversion10/1 -> Data/1
  Add2/1 -> Divide9/1
  Divide9/1 -> Add5/1
  Constant10/1 -> Divide6/2
  HighByte/1 -> Divide6/1
  Add5/1 -> Data Type Conversion10/1
  LowByte/1 -> Add2/1
  Divide6/1 -> Add2/2

== system EPT/Foreground_TimeBase_5ms/CAN/CAN3_exec/PWCU_GENERATOR/PWCU/PWCU1_Rx/Convert_Byte2Data ==
  HighByte : Inport
  LowByte : Inport  Port=2
  Offset : Inport  Port=3
  Factor : Inport  Port=4
  Add2 : Sum
  Add5 : Sum
  Constant10 : Constant  Value=256
  Data Type Conversion10 : DataTypeConversion  OutDataTypeStr=double
  Divide6 : Product  Inputs=**
  Divide9 : Product  Inputs=**
  Data : Outport  VectorParamsAs1DForOutWhenUnconnected=off
  wires:
  Divide6/1 -> Add2/2
  LowByte/1 -> Add2/1
  Add5/1 -> Data Type Conversion10/1
  HighByte/1 -> Divide6/1
  Constant10/1 -> Divide6/2
  Divide9/1 -> Add5/1
  Add2/1 -> Divide9/1
  Data Type Conversion10/1 -> Data/1
  Factor/1 -> Divide9/2
  Offset/1 -> Add5/2

== system EPT/Foreground_TimeBase_5ms/CAN/CAN3_exec/PWCU_GENERATOR/PWCU/PWCU1_Rx/Convert_Byte2Data1 ==
  HighByte : Inport
  LowByte : Inport  Port=2
  Offset : Inport  Port=3
  Factor : Inport  Port=4
  Add2 : Sum
  Add5 : Sum
  Constant10 : Constant  Value=256
  Data Type Conversion10 : DataTypeConversion  OutDataTypeStr=double
  Divide6 : Product  Inputs=**
  Divide9 : Product  Inputs=**
  Data : Outport  VectorParamsAs1DForOutWhenUnconnected=off
  wires:
  Divide6/1 -> Add2/2
  LowByte/1 -> Add2/1
  Add5/1 -> Data Type Conversion10/1
  HighByte/1 -> Divide6/1
  Constant10/1 -> Divide6/2
  Divide9/1 -> Add5/1
  Add2/1 -> Divide9/1
  Data Type Conversion10/1 -> Data/1
  Factor/1 -> Divide9/2
  Offset/1 -> Add5/2

== system EPT/Foreground_TimeBase_5ms/CAN/CAN3_exec/PWCU_GENERATOR/PWCU/PWCU1_Rx/Convert_Byte2Data2 ==
  HighByte : Inport
  LowByte : Inport  Port=2
  Offset : Inport  Port=3
  Factor : Inport  Port=4
  Add2 : Sum
  Add5 : Sum
  Constant10 : Constant  Value=256
  Data Type Conversion10 : DataTypeConversion  OutDataTypeStr=double
  Divide6 : Product  Inputs=**
  Divide9 : Product  Inputs=**
  Data : Outport  VectorParamsAs1DForOutWhenUnconnected=off
  wires:
  Divide6/1 -> Add2/2
  LowByte/1 -> Add2/1
  Add5/1 -> Data Type Conversion10/1
  HighByte/1 -> Divide6/1
  Constant10/1 -> Divide6/2
  Divide9/1 -> Add5/1
  Add2/1 -> Divide9/1
  Data Type Conversion10/1 -> Data/1
  Factor/1 -> Divide9/2
  Offset/1 -> Add5/2

== system EPT/Foreground_TimeBase_5ms/CAN/CAN3_exec/PWCU_GENERATOR/PWCU/PWCU1_Tx/Convert_Data2Byte ==
  Data : Inport
  Factor : Inport  Port=2
  Offset : Inport  Port=3
  Add1 : Sum
  Bitwise Operator : simulink/Logic and Bit Operations/Bitwise Operator  logicop=AND  UseBitMask=on  BitMask=bin2dec('1111111100000000')  BitMaskRealWorld=Stored Integer
  Bitwise Operator1 : simulink/Logic and Bit Operations/Bitwise Operator  logicop=AND  UseBitMask=on  BitMask=bin2dec('0000000011111111')  BitMaskRealWorld=Stored Integer
  Constant : Constant
  Data Type Conversion1 : DataTypeConversion  OutDataTypeStr=uint16
  Divide1 : Product  Inputs=*/
  Divide2 : Product  Inputs=**
  Shift Arithmetic : ArithShift  BitShiftNumber=8  BitShiftDirection=Right
  HighByte : Outport  VectorParamsAs1DForOutWhenUnconnected=off
  LowByte : Outport  Port=2  VectorParamsAs1DForOutWhenUnconnected=off
  wires:
  Divide2/1 -> Data Type Conversion1/1
  Data/1 -> Add1/1
  Add1/1 -> Divide2/1
  Data Type Conversion1/1 -> Bitwise Operator1/1, Bitwise Operator/1
  Bitwise Operator1/1 -> LowByte/1
  Shift Arithmetic/1 -> HighByte/1
  Offset/1 -> Add1/2
  Bitwise Operator/1 -> Shift Arithmetic/1
  Factor/1 -> Divide1/2
  Divide1/1 -> Divide2/2
  Constant/1 -> Divide1/1

== system EPT/Foreground_TimeBase_5ms/CAN/CAN3_exec/PWCU_GENERATOR/PWCU/PWCU1_Tx/Convert_Data2Byte1 ==
  Data : Inport
  Factor : Inport  Port=2
  Offset : Inport  Port=3
  Add1 : Sum
  Bitwise Operator : simulink/Logic and Bit Operations/Bitwise Operator  logicop=AND  UseBitMask=on  BitMask=bin2dec('1111111100000000')  BitMaskRealWorld=Stored Integer
  Bitwise Operator1 : simulink/Logic and Bit Operations/Bitwise Operator  logicop=AND  UseBitMask=on  BitMask=bin2dec('0000000011111111')  BitMaskRealWorld=Stored Integer
  Constant : Constant
  Data Type Conversion1 : DataTypeConversion  OutDataTypeStr=uint16
  Divide1 : Product  Inputs=*/
  Divide2 : Product  Inputs=**
  Shift Arithmetic : ArithShift  BitShiftNumber=8  BitShiftDirection=Right
  HighByte : Outport  VectorParamsAs1DForOutWhenUnconnected=off
  LowByte : Outport  Port=2  VectorParamsAs1DForOutWhenUnconnected=off
  wires:
  Divide2/1 -> Data Type Conversion1/1
  Data/1 -> Add1/1
  Add1/1 -> Divide2/1
  Data Type Conversion1/1 -> Bitwise Operator1/1, Bitwise Operator/1
  Bitwise Operator1/1 -> LowByte/1
  Shift Arithmetic/1 -> HighByte/1
  Offset/1 -> Add1/2
  Bitwise Operator/1 -> Shift Arithmetic/1
  Factor/1 -> Divide1/2
  Divide1/1 -> Divide2/2
  Constant/1 -> Divide1/1

== system EPT/Foreground_TimeBase_5ms/CAN/CAN3_exec/PWCU_GENERATOR/PWCU/PWCU2_Tx/Convert_Data2Byte ==
  Data : Inport
  Factor : Inport  Port=2
  Offset : Inport  Port=3
  Add1 : Sum
  Bitwise Operator : simulink/Logic and Bit Operations/Bitwise Operator  logicop=AND  UseBitMask=on  BitMask=bin2dec('1111111100000000')  BitMaskRealWorld=Stored Integer
  Bitwise Operator1 : simulink/Logic and Bit Operations/Bitwise Operator  logicop=AND  UseBitMask=on  BitMask=bin2dec('0000000011111111')  BitMaskRealWorld=Stored Integer
  Constant : Constant
  Data Type Conversion1 : DataTypeConversion  OutDataTypeStr=uint16
  Divide1 : Product  Inputs=*/
  Divide2 : Product  Inputs=**
  Shift Arithmetic : ArithShift  BitShiftNumber=8  BitShiftDirection=Right
  HighByte : Outport  VectorParamsAs1DForOutWhenUnconnected=off
  LowByte : Outport  Port=2  VectorParamsAs1DForOutWhenUnconnected=off
  wires:
  Divide2/1 -> Data Type Conversion1/1
  Data/1 -> Add1/1
  Add1/1 -> Divide2/1
  Data Type Conversion1/1 -> Bitwise Operator1/1, Bitwise Operator/1
  Bitwise Operator1/1 -> LowByte/1
  Shift Arithmetic/1 -> HighByte/1
  Offset/1 -> Add1/2
  Bitwise Operator/1 -> Shift Arithmetic/1
  Factor/1 -> Divide1/2
  Divide1/1 -> Divide2/2
  Constant/1 -> Divide1/1

== system EPT/Foreground_TimeBase_5ms/CAN/CAN3_exec/PWCU_GENERATOR/PWCU/PWCU2_Tx/Convert_Data2Byte1 ==
  Data : Inport
  Factor : Inport  Port=2
  Offset : Inport  Port=3
  Add1 : Sum
  Bitwise Operator : simulink/Logic and Bit Operations/Bitwise Operator  logicop=AND  UseBitMask=on  BitMask=bin2dec('1111111100000000')  BitMaskRealWorld=Stored Integer
  Bitwise Operator1 : simulink/Logic and Bit Operations/Bitwise Operator  logicop=AND  UseBitMask=on  BitMask=bin2dec('0000000011111111')  BitMaskRealWorld=Stored Integer
  Constant : Constant
  Data Type Conversion1 : DataTypeConversion  OutDataTypeStr=uint16
  Divide1 : Product  Inputs=*/
  Divide2 : Product  Inputs=**
  Shift Arithmetic : ArithShift  BitShiftNumber=8  BitShiftDirection=Right
  HighByte : Outport  VectorParamsAs1DForOutWhenUnconnected=off
  LowByte : Outport  Port=2  VectorParamsAs1DForOutWhenUnconnected=off
  wires:
  Divide2/1 -> Data Type Conversion1/1
  Data/1 -> Add1/1
  Add1/1 -> Divide2/1
  Data Type Conversion1/1 -> Bitwise Operator1/1, Bitwise Operator/1
  Bitwise Operator1/1 -> LowByte/1
  Shift Arithmetic/1 -> HighByte/1
  Offset/1 -> Add1/2
  Bitwise Operator/1 -> Shift Arithmetic/1
  Factor/1 -> Divide1/2
  Divide1/1 -> Divide2/2
  Constant/1 -> Divide1/1
